simulink model "basesoft"  (R2025b)
settings: configuration reference "MCConfiguration" (kept outside this file)
settings Model: DataDictionary=embeddedBoard_common.sldd  Creator=rpumpo  LastModifiedBy=rpumpo
settings ConfigSetRef: SourceName=MCConfiguration

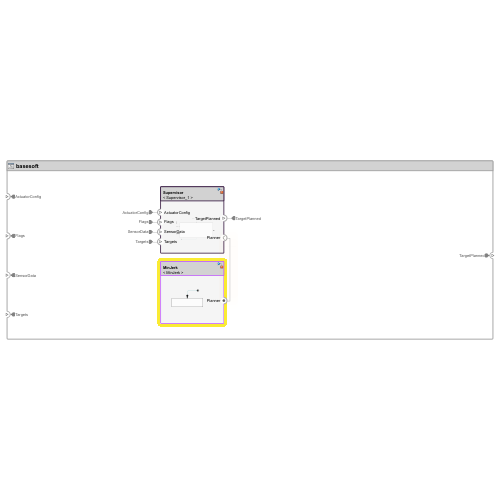
[thumbnail: Simulink's stored preview of the top-level diagram]
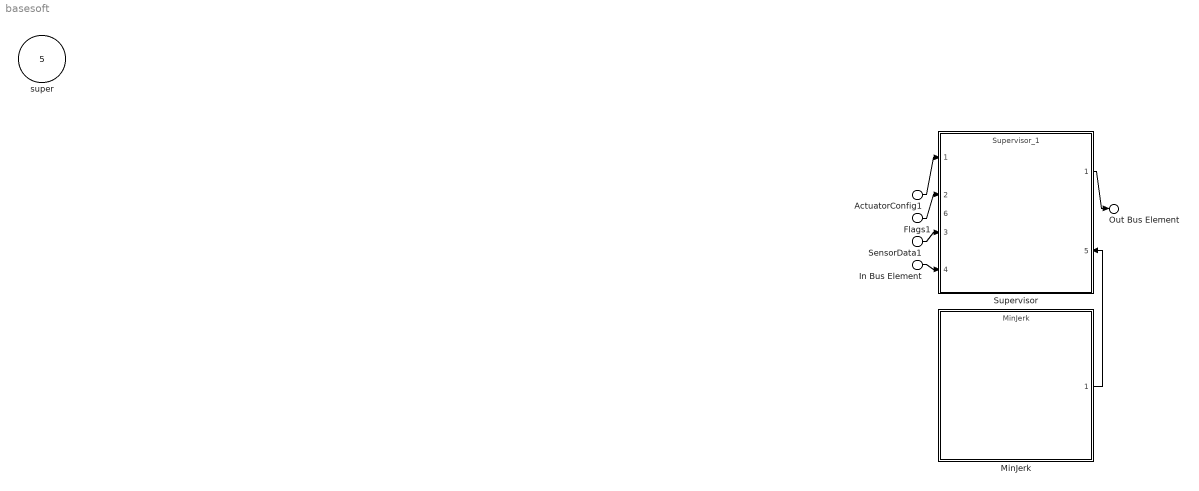
== system basesoft ==
  ActuatorConfig1 : Inport  PortName=ActuatorConfig
  Flags1 : Inport  Port=2  PortName=Flags
  SensorData1 : Inport  Port=3  PortName=SensorData
  In Bus Element : Inport  Port=4  PortName=Targets
  super : Inport  Port=5  OutputFunctionCall=on
  MinJerk : ModelReference  ModelNameDialog=MinJerk.slx  SimulationMode=Normal  ScheduleRates=on  ModelReferenceVersion=1.12
      settings: PortSchema="{\"entries\":[{\"content\":{\"headerSize\":38,\"margin\":15,\"minimumSpacing\":25,\"sides\":[{\"content\":{},\"type\":\"ConnectorPlacement.EquallySpacedRectSide\",\"uuid\":\"60267e4b-699d-4299-a7d3-7d1fc4f5da23\"},{\"content\":{\"connectorIds\":[\"Out1\"],\"side\":\"RIGHT\"},\"type\":\"ConnectorPlacement.EquallySpacedRectSide\",\"uuid\":\"a1e24c49-5c27-4ee4-836e-f88f3fe2b9d9\"},{\"content\":{\"side\":\"TOP\"},\"type\":\"ConnectorPlacement.EquallySpacedRectSide\",\"uuid\":\"5ae85150-b5c9-4175-9e2e-13fbe12c1c70\"}]},\"type\":\"ConnectorPlacement.EquallySpacedConnector\",\"uuid\":\"d6d3337e-45b6-4923-9a42-676322c3db2b\"}],\"packageUris\":[\"http://schema.mathworks.com/mf0/Connector/R2020b\"],\"version\":\"1.0\"}"
  Supervisor : ModelReference  ModelNameDialog=Supervisor_1  SimulationMode=Normal  ScheduleRates=on  CachedPortDiscreteRates=[0.001]  ModelReferenceVersion=1.16
      settings: PortSchema="{\"entries\":[{\"content\":{\"headerSize\":38,\"margin\":15,\"minimumSpacing\":25,\"sides\":[{\"content\":{\"connectorIds\":[\"In1\",\"In2\",\"In3\",\"In4\"]},\"type\":\"ConnectorPlacement.EquallySpacedRectSide\",\"uuid\":\"60267e4b-699d-4299-a7d3-7d1fc4f5da23\"},{\"content\":{\"connectorIds\":[\"Out1\",\"In5\"],\"side\":\"RIGHT\"},\"type\":\"ConnectorPlacement.EquallySpacedRectSide\",\"uuid\":\"a1e24c49-5c27-4ee4-836e-f88f3fe2b9d9\"},{\"content\":{\"side\":\"TOP\"},\"type\":\"ConnectorPlacement.EquallySpacedRectSide\",\"uuid\":\"5ae85150-b5c9-4175-9e2e-13fbe12c1c70\"},{\"content\":{\"connectorIds\":[\"In6\"],\"side\":\"HIDDEN\"},\"type\":\"ConnectorPlacement.EquallySpacedRectSide\",\"uuid\":\"7466e11e-5ec6-4b50-bee6-5b0ad19b64b0\"}]},\"type\":\"ConnectorPlacement.EquallySpacedConnector\",\"uuid\":\"d6d3337e-45b6-4923-9a42-676322c3db2b\"}],\"packageUris\":[\"http://schema.mathworks.com/mf0/Connector/R2020b\"],\"version\":\"1.0\"}"
  Out Bus Element : Outport  PortName=TargetPlanned
  wires:
  ActuatorConfig1/1 -> Supervisor/1
  Flags1/1 -> Supervisor/2
  MinJerk/1 -> Supervisor/5
  SensorData1/1 -> Supervisor/3
  In Bus Element/1 -> Supervisor/4
  Supervisor/1 -> Out Bus Element/1
